simulink model "Check_wind2body_axis_transformation"  (R2016a)
settings: Solver=ode4  StartTime=0.0  StopTime=10.0  FixedStep=0.001  RelTol=1e-3
libraries: aerolibconvert2 x2
settings Model: Creator=PD Banneheka  LastModifiedBy=PD Banneheka
settings GRTTargetCC: GeneratePreprocessorConditionals=Use local settings

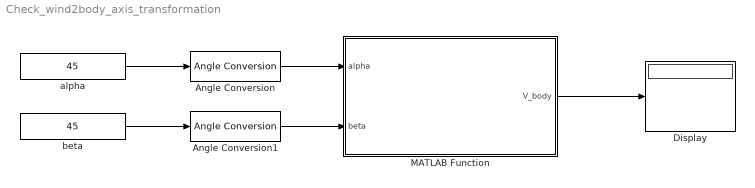
== system Check_wind2body_axis_transformation ==
  Angle Conversion : aerolibconvert2/Angle Conversion  IU=deg  OU=rad
  Angle Conversion1 : aerolibconvert2/Angle Conversion  IU=deg  OU=rad
  Display : Display
  MATLAB Function : MATLAB Function  TreatAsAtomicUnit=on
  alpha : Constant  Value=45
  beta : Constant  Value=45
  wires:
  MATLAB Function/1(V_body) -> Display/1
  Angle Conversion1/1 -> MATLAB Function/2(beta)
  Angle Conversion/1 -> MATLAB Function/1(alpha)
  alpha/1 -> Angle Conversion/1
  beta/1 -> Angle Conversion1/1

== matlab function Check_wind2body_axis_transformation/MATLAB Function ==
  data: alpha input; V_body output; beta input
function V_body = fcn(alpha,beta)

% According to Cook (page 21): (phi,theta,psi) = (0,alpha,-beta)
phi = 0;
theta = alpha;
psi = -beta;

% NASA transformation equations
theta1 = psi;
theta2 = theta;
theta3 = phi;

q0 = +sin(theta1/2)*sin(theta2/2)*sin(theta3/2)+cos(theta1/2)*cos(theta2/2)*cos(theta3/2);
q1 = -sin(theta1/2)*sin(theta2/2)*cos(theta3/2)+sin(theta3/2)*cos(theta1/2)*cos(theta2/2);
q2 = +sin(theta1/2)*sin(theta3/2)*cos(theta2/2)+sin(theta2/2)*cos(theta1/2)*cos(theta3/2);
q3 = +sin(theta1/2)*cos(theta2/2)*cos(theta3/2)-sin(theta2/2)*sin(theta3/2)*cos(theta1/2);

E = [  -q1     q0      -q3     q2
        -q2     q3      q0      -q1
        -q3     -q2     q1      q0  ];
    
E_dash = [     -q1     q0      q3      -q2
                -q2     -q3     q0      q1
                -q3     q2      -q1     q0  ];
            
A_b2w = E*transpose(E_dash);

V0 = [  30
        0
        0   ];
    
V_body = transpose(A_b2w)*V0;
